simulink model "ES105A_StHlthSigNormn"  (R2013b)
settings: Solver=FixedStepDiscrete  SolverMode=SingleTasking  StartTime=0.0  StopTime=1  FixedStep=0.002  RelTol=1e-3
undefined symbols (not defined in the file): ARCHGLBPRM_FLOATZEROTHD_ULS_F32, CurrMeasCorrlnMaxErrCurr, CURRMOTSUMDIVBYZEROPROTNVAL_AMPR_F32, DIGTQDIVBYZEROPROTNVAL_HWNWTMTR_F32, DutyCycThermProtnDutyCycFildThd, EcuTMeasRngDiagcMax, EcuTMeasRngDiagcMin, EotLrngAuthyStrtLrn, FRICESTIMNDIVBYZEROPROTNVAL_HWNWTMTR_F32, HLTH0PERC_CNT_U08, HLTH100PERC_CNT_F32, HLTH100PERC_CNT_U08, HLTH50PERC_CNT_U08, HwTqCorrlnChATraSumSetFltThd, HwTqCorrlnChBTraSumSetFltThd, HWTQIDPTSIG_CNT_U08, MOTAG2MEAS_VALMAXERR_VOLTSQD_F32, MOTAG2MEAS_VALMINERR_VOLTSQD_F32, MOTAGCORRLN_MOTAGCORRLNERRTHD_MOTREVELEC_U0P16, MotDrvDiagcErrThd, MOTPOS2DIVBYZEROPROTNVAL2_VOLTSQD_F32, MOTPOS2DIVBYZEROPROTNVAL_VOLTSQD_F32, MOTPOSNERRDIVBYZEROPROTNVAL_MOTREV_U16, MOTPOSNERRZEROTHD_MOTREV_U0P16, NtcNr1, NtcSts1, PHAVLTGDIVBYZEROPROTNVAL_NANOSEC_F32, SigQlfr1, STHLTHSCAGFAC_CNT_F32, StHlthSigNormnAbsltMotPosDifStHlthDiagThd, StHlthSigNormnCurrMotSumStHlthDiagThd, StHlthSigNormnDigTqStHlthDiagThd, StHlthSigNormnDutyCycFltLimThd, StHlthSigNormnHiCtrlrT, StHlthSigNormnIdptSigStHlthSca, StHlthSigNormnLoCtrlrT, StHlthSigNormnMaxFricThd, StHlthSigNormnMinRackTrvlLim, StHlthSigNormnMotPosStHlthDiagThd, StHlthSigNormnMotVelCal, StHlthSigNormnPhaInfoStHlthDiagThd, StHlthSigNormnStHlthCorrlnErr, StHlthSigNormnStHlthCurrMotSum, StHlthSigNormnStHlthPhaInfo, StHlthSigNormnValMaxStHlthErr, StHlthSigNormnValMinStHlthErr, StHlthSigNormnWhlImbRejctnThd, SysGlbPrmMotPoleCnt, TSTHLTH0PERC_CNT_U08, u2, u3, u4, VLTGSTHLTH0PERC_CNT_U08
libraries: NxtrLim x39, simulink x33, NxtrAbslt x4
(part 2 of 10)

== system ES105A_StHlthSigNormn/StHlthSigNormn/StHlthSigNormnInit1/Motror Angle Threshold Calc ==
  note: MotAgCorrlnErrThd_p32
  note: p16
  note: p0
  note: 2^16 is max resolution
      | of 1/MotPoleCnt that won't
      | overflow u32
  note: MotPoleCnt.Max = 12
      | MotPoleCnt.Min = 2
  note: The MotAgA vs MotAgB comparison diagnostic
      | in this FDD compares MotAg signals in MotRev.
      | The safety consideration for these comparisons
      | is in MotRevElec.  Therefore the error threshold
      | has to be converted to MotRev via the following
      | relationship:
      |
      | MotRev * Np/2 = MotElec
      | MotRevElec * 2/Np = MotRev
  note: 1/MotPole_p16.Max = 32768
      | 1/MotPole_p16.Min = 5461
  note: 1 as p16
  note: MotAgCorrlnErrThd_p16
  1 as 2^16 : Constant  OutDataTypeStr=uint32
  CopyRight2 : Subsystem  Description=|  mask(Copyright Information){none=on}
      | Copyright info block.                                               
      |                                                                     
      | Place copyright information at the top of every subsystem in design.
      mask prompts: none "No parameters"
      mask help: Place copyright information at the top of every subsystem in design.
      mask Display:
      | NxtrConf = 'Nexteer Confidential';
      | 
      | sys = bdroot; %handle for the current model ("system")
      | first = get_param(sys,'Created');
      | if(isempty(first))
      |     first = datestr(now,'yyyy');
      | else
      |     first = first(end-3:end);  %year is last four digits
      | end
      | 
      | last = get_param(sys,'LastModifiedDate');
      | if isempty(last)
      |     last = datestr(now,'yyyy');
      | else
      |     last = last(end-3:end);
      | end
      | 
      | if strcmp(first,last)
      |     fprintf('%s -- Copyright %s Nexteer',NxtrConf,first)
      | else
      |     fprintf('%s -- %s%s- %s Nexteer',NxtrConf,char(169),first,last)
      | end
  Data Type Conversion{,1..4} (5 alike) : DataTypeConversion  OutDataTypeStr=uint32
  Data Type Conversion5 : DataTypeConversion  OutDataTypeStr=uint16
  Divide : Product  Inputs=*/
  Gain : Gain  Gain=-1  OutDataTypeStr=int8
  MOTAGCORRLNERRTHD_MOTREVELEC_U0P16 Data Type Max = 65535 : Constant  Value=MOTAGCORRLN_MOTAGCORRLNERRTHD_MOTREVELEC_U0P16
  MotAgCorrlnErrThd : DataStoreWrite  DataStoreName=MotAgCorrlnErrThd
  Numerator Precision : Constant  Value=16  OutDataTypeStr=int8
  Product : Product  Inputs=3
  Shift Arithmetic : ArithShift  BitShiftNumberSource=Input port  BitShiftNumber=16
      settings: InputPortMap=u0,p1
  Shift Arithmetic1 : ArithShift  BitShiftNumberSource=Input port  BitShiftNumber=16
      settings: InputPortMap=u0,p1
  SysGlbPrmMotPoleCnt : Constant  Value=SysGlbPrmMotPoleCnt
  Two Max = 2 : Constant  Value=2  OutDataTypeStr=uint32
  wires:
  SysGlbPrmMotPoleCnt/1 -> Data Type Conversion/1
  1 as 2^16/1 -> Shift Arithmetic1/1
  Shift Arithmetic1/1 -> Data Type Conversion1/1
  Data Type Conversion/1 -> Divide/2
  MOTAGCORRLNERRTHD_MOTREVELEC_U0P16 Data Type Max = 65535/1 -> Data Type Conversion2/1
  Two Max = 2/1 -> Data Type Conversion3/1
  Divide/1 -> Product/3
  Product/1 -> Data Type Conversion4/1
  Data Type Conversion3/1 -> Product/2
  Data Type Conversion2/1 -> Product/1
  Data Type Conversion5/1 -> MotAgCorrlnErrThd/1
  Data Type Conversion4/1 -> Shift Arithmetic/1
  Shift Arithmetic/1 -> Data Type Conversion5/1
  Numerator Precision/1 -> Gain/1, Shift Arithmetic/2
  Gain/1 -> Shift Arithmetic1/2
  Data Type Conversion1/1 -> Divide/1

== system ES105A_StHlthSigNormn/StHlthSigNormn/UpdRawSig/ EOT Impact Counter ==
  "HwAuthy " : Inport
  HwAg : Inport  Port=2
  RackLimrEotSig1Avl : Inport  Port=3
  HwAgEotCw : Inport  Port=4
  MotVelCrf : Inport  Port=5
  RackLimrEotSig0Avl : Inport  Port=6
  HwAgEotCcw : Inport  Port=7
  "Case:{}" : ActionPort  ActionType=case
  Constant : Constant  Value=EotLrngAuthyStrtLrn
  CopyRight2 : Subsystem  Description=|  mask(Copyright Information){none=on}
      | Copyright info block.                                               
      |                                                                     
      | Place copyright information at the top of every subsystem in design.
      mask prompts: none "No parameters"
      mask help: Place copyright information at the top of every subsystem in design.
      mask Display:
      | NxtrConf = 'Nexteer Confidential';
      | 
      | sys = bdroot; %handle for the current model ("system")
      | first = get_param(sys,'Created');
      | first = first(end-3:end);  %year is last four digits
      | 
      | last = get_param(sys,'LastModifiedDate');
      | if isempty(last)
      |     last = datestr(now,'yyyy');
      | else
      |     last = last(end-3:end);
      | end
      | 
      | if strcmp(first,last)
      |     fprintf('%s -- Copyright %s Nexteer',NxtrConf,first)
      | else
      |     fprintf('%s -- %s%s- %s Nexteer',NxtrConf,char(169),first,last)
      | end
  Data Store Read : DataStoreRead  DataStoreName=EotImpctCntr
  If : If  IfExpression=u1
  If Action Subsystem : Subsystem  TreatAsAtomicUnit=on
  If Action Subsystem1 : Subsystem  TreatAsAtomicUnit=on
  LimStat_u2 : NxtrLim/LimStat_u08  LoLim=EotImpctStHlth.EngMin  HiLim=EotImpctStHlth.EngMax
      settings: AttributesFormatString=|
      | Low Limit: %<LoLim>
      | High Limit:%<HiLim>
  Relational Operator : RelationalOperator  Operator=>  OutDataTypeStr=boolean
  EotImpctStHlth : Outport
  wires:
  "HwAuthy "/1 -> Relational Operator/1
  Constant/1 -> Relational Operator/2
  Relational Operator/1 -> If/1
  If/1 -> If Action Subsystem/Action
  HwAg/1 -> If Action Subsystem/1(HwAg)
  If/2 -> If Action Subsystem1/Action
  RackLimrEotSig1Avl/1 -> If Action Subsystem/5(RackLimrEotSig1Avl)
  RackLimrEotSig0Avl/1 -> If Action Subsystem/2(RackLimrEotSig0Avl)
  HwAgEotCw/1 -> If Action Subsystem/6(HwAgEotCw)
  MotVelCrf/1 -> If Action Subsystem/3(MotVelCrf)
  HwAgEotCcw/1 -> If Action Subsystem/4(HwAgEotCcw)
  Data Store Read/1 -> LimStat_u2/1
  LimStat_u2/1 -> EotImpctStHlth/1

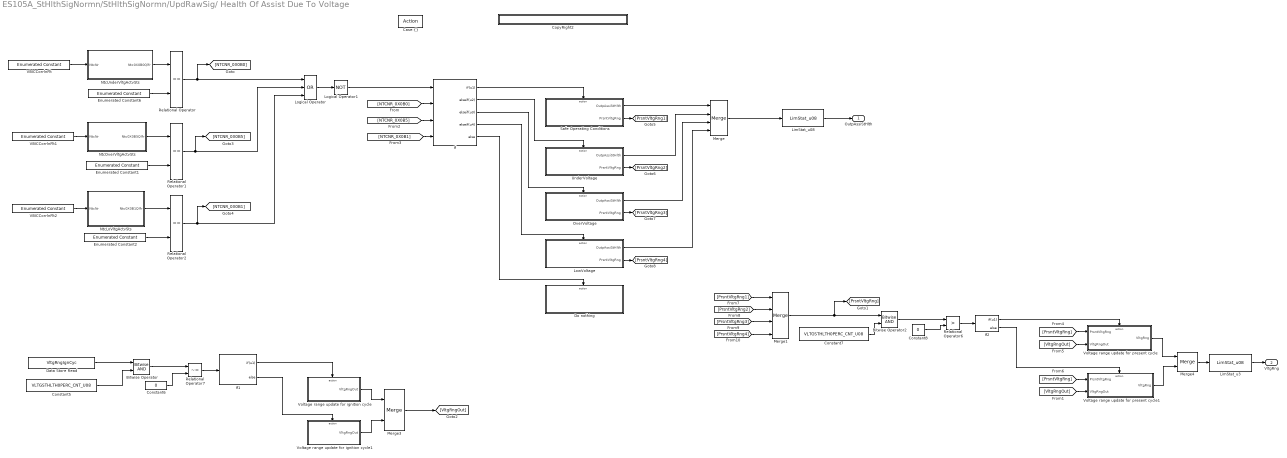
== system ES105A_StHlthSigNormn/StHlthSigNormn/UpdRawSig/ Health Of Assist Due To Voltage ==
  "Case:{}" : ActionPort  ActionType=case
  Bitwise Operator : simulink/Logic and Bit Operations/Bitwise Operator  logicop=AND  UseBitMask=off  NumInputPorts=2  BitMask=bin2dec('11011001')  BitMaskRealWorld=Stored Integer
  Bitwise Operator2 : simulink/Logic and Bit Operations/Bitwise Operator  logicop=AND  UseBitMask=off  NumInputPorts=2  BitMask=bin2dec('11011001')  BitMaskRealWorld=Stored Integer
  Constant5 : Constant  Value=VLTGSTHLTH0PERC_CNT_U08
  Constant6 : Constant  Value=0  OutDataTypeStr=uint8
      settings: AttributesFormatString=%<OutDataTypeStr>
  Constant7 : Constant  Value=VLTGSTHLTH0PERC_CNT_U08
  Constant8 : Constant  Value=0  OutDataTypeStr=uint8
      settings: AttributesFormatString=%<OutDataTypeStr>
  CopyRight2 : Subsystem  Description=|  mask(Copyright Information){none=on}
      | Copyright info block.                                               
      |                                                                     
      | Place copyright information at the top of every subsystem in design.
      mask prompts: none "No parameters"
      mask help: Place copyright information at the top of every subsystem in design.
      mask Display:
      | NxtrConf = 'Nexteer Confidential';
      | 
      | sys = bdroot; %handle for the current model ("system")
      | first = get_param(sys,'Created');
      | first = first(end-3:end);  %year is last four digits
      | 
      | last = get_param(sys,'LastModifiedDate');
      | if isempty(last)
      |     last = datestr(now,'yyyy');
      | else
      |     last = last(end-3:end);
      | end
      | 
      | if strcmp(first,last)
      |     fprintf('%s -- Copyright %s Nexteer',NxtrConf,first)
      | else
      |     fprintf('%s -- %s%s- %s Nexteer',NxtrConf,char(169),first,last)
      | end
  Data Store Read : DataStoreRead  DataStoreName=VltgRngIgnCyc
  Do nothing : Subsystem
  Enumerated Constant1 : simulink/Sources/Enumerated Constant  OutDataTypeStr=Enum: SigQlfr1  Value=SigQlfr1.SIGQLFR_FAILD  SampleTime=inf
  Enumerated Constant2 : simulink/Sources/Enumerated Constant  OutDataTypeStr=Enum: SigQlfr1  Value=SigQlfr1.SIGQLFR_FAILD  SampleTime=inf
  Enumerated Constant6 : simulink/Sources/Enumerated Constant  OutDataTypeStr=Enum: SigQlfr1  Value=SigQlfr1.SIGQLFR_FAILD  SampleTime=inf
  If : If  NumInputs=4  IfExpression=u1  ElseIfExpressions=u2,u3,u4
  If1 : If  IfExpression=u1
  If2 : If  IfExpression=u1
  LimStat_u08 : NxtrLim/LimStat_u08  LoLim=OutpAssiStHlth.EngMin  HiLim=OutpAssiStHlth.EngMax
      settings: AttributesFormatString=|
      | Low Limit: %<LoLim>
      | High Limit:%<HiLim>
  LimStat_u3 : NxtrLim/LimStat_u08  LoLim=VltgRng.EngMin  HiLim=VltgRng.EngMax
      settings: AttributesFormatString=|
      | Low Limit: %<LoLim>
      | High Limit:%<HiLim>
  Logical Operator : Logic  RequirementInfo={'linktype_rmi_doors' '0001022c (/ESG Group/FDD Module Requirements/EA4 Specific/ES105A_StHlthSigNormn)' '#ES105A_50' 'true' 'REQ: ES105A_50' '' } %GIDa_9a5ea61a_ea12_4910_a0fe_06a0e1905550  Operator=OR  Inputs=3  AllPortsSameDT=off  OutDataTypeStr=boolean
  Logical Operator1 : Logic  RequirementInfo={'linktype_rmi_doors' '0001022c (/ESG Group/FDD Module Requirements/EA4 Specific/ES105A_StHlthSigNormn)' '#ES105A_50' 'true' 'REQ: ES105A_50' '' } %GIDa_f3dc77f5_d391_4300_bddf_a50a41924f40  Operator=NOT  AllPortsSameDT=off  OutDataTypeStr=boolean
  LowVoltage : Subsystem  RequirementInfo={'linktype_rmi_doors' '0001022c (/ESG Group/FDD Module Requirements/EA4 Specific/ES105A_StHlthSigNormn)' '#ES105A_53' 'true' 'REQ: ES105A_53' '' } %GIDa_506e871b_8543_4634_a577_67c158e429f9
  Merge : Merge  Inputs=4
  Merge1 : Merge  Inputs=4
  Merge3 : Merge
  Merge4 : Merge
  NtcLoVltgActvSts : Subsystem  RequirementInfo={} %GIDa_d5ea79d0_4b56_4532_81dc_37f5b337e086  TreatAsAtomicUnit=on  mask(GetNTC){}
      mask help: GetNTC library block
      settings: RTWSystemCode=Inline
  NtcOverVltgActvSts : Subsystem  RequirementInfo={} %GIDa_e1e8ebde_c4f9_4f8d_a1e3_0543f63840ce  TreatAsAtomicUnit=on  mask(GetNTC){}
      mask help: GetNTC library block
      settings: RTWSystemCode=Inline
  NtcUnderVltgActvSts : Subsystem  RequirementInfo={} %GIDa_9b87baab_3980_45fe_8d54_a3baaaee6b6f  TreatAsAtomicUnit=on  mask(GetNTC){}
      mask help: GetNTC library block
      settings: RTWSystemCode=Inline
  OverVoltage : Subsystem  RequirementInfo={'linktype_rmi_doors' '0001022c (/ESG Group/FDD Module Requirements/EA4 Specific/ES105A_StHlthSigNormn)' '#ES105A_52' 'true' 'REQ: ES105A_52' '' } %GIDa_cd3c8530_bf41_482a_97a1_1e49fef579f6
  Relational Operator : RelationalOperator  Operator===  OutDataTypeStr=boolean
  Relational Operator1 : RelationalOperator  Operator===  OutDataTypeStr=boolean
  Relational Operator2 : RelationalOperator  Operator===  OutDataTypeStr=boolean
  Relational Operator6 : RelationalOperator  Operator=>  OutDataTypeStr=boolean
  Relational Operator7 : RelationalOperator  Operator=~=  OutDataTypeStr=boolean
  Safe Operating Conditions : Subsystem  RequirementInfo={'linktype_rmi_doors' '0001022c (/ESG Group/FDD Module Requirements/EA4 Specific/ES105A_StHlthSigNormn)' '#ES105A_50' 'true' 'REQ: ES105A_50' '' } %GIDa_08090837_8a60_4bda_aaf5_7b407a469d1b
  UnderVoltage : Subsystem  RequirementInfo={'linktype_rmi_doors' '0001022c (/ESG Group/FDD Module Requirements/EA4 Specific/ES105A_StHlthSigNormn)' '#ES105A_51' 'true' 'REQ: ES105A_51' '' } %GIDa_8bbe1a5e_3828_4897_9c76_848f46c9da8f
  VBICCorrlnFlt : simulink/Sources/Enumerated Constant  RequirementInfo={'linktype_rmi_doors' '0001022c (/ESG Group/FDD Module Requirements/EA4 Specific/ES105A_StHlthSigNormn)' '#ES105A_15' 'true' 'REQ: ES105A_15' '' } %GIDa_abcae5bb_89f4_46e7_b061_adbd8ff599e2  OutDataTypeStr=Enum: NtcNr1  Value=NtcNr1.NTCNR_0X0B0  SampleTime=inf
  VBICCorrlnFlt1 : simulink/Sources/Enumerated Constant  RequirementInfo={'linktype_rmi_doors' '0001022c (/ESG Group/FDD Module Requirements/EA4 Specific/ES105A_StHlthSigNormn)' '#ES105A_15' 'true' 'REQ: ES105A_15' '' } %GIDa_5d58c9da_5328_4e21_8197_5deed1f7c707  OutDataTypeStr=Enum: NtcNr1  Value=NtcNr1.NTCNR_0X0B5  SampleTime=inf
  VBICCorrlnFlt2 : simulink/Sources/Enumerated Constant  RequirementInfo={'linktype_rmi_doors' '0001022c (/ESG Group/FDD Module Requirements/EA4 Specific/ES105A_StHlthSigNormn)' '#ES105A_15' 'true' 'REQ: ES105A_15' '' } %GIDa_7ebd8b39_32ce_4267_96b1_a79cedaf356f  OutDataTypeStr=Enum: NtcNr1  Value=NtcNr1.NTCNR_0X0B1  SampleTime=inf
  Voltage range update for ignition cycle : Subsystem  RequirementInfo={'linktype_rmi_doors' '0001022c (/ESG Group/FDD Module Requirements/EA4 Specific/ES105A_StHlthSigNormn)' '#ES105A_54' 'true' 'REQ: ES105A_54' '' } %GIDa_370b8f01_3508_495b_a218_3f1e9e3ef072  TreatAsAtomicUnit=on
  Voltage range update for ignition cycle1 : Subsystem  RequirementInfo={'linktype_rmi_doors' '0001022c (/ESG Group/FDD Module Requirements/EA4 Specific/ES105A_StHlthSigNormn)' '#ES105A_54' 'true' 'REQ: ES105A_54' '' } %GIDa_2af8c5ef_4773_490c_9b01_2c7f0f74e411  TreatAsAtomicUnit=on
  "Voltage range update for present cycle " : Subsystem  RequirementInfo={'linktype_rmi_doors' '0001022c (/ESG Group/FDD Module Requirements/EA4 Specific/ES105A_StHlthSigNormn)' '#ES105A_54' 'true' 'REQ: ES105A_54' '' } %GIDa_0b645a7d_a4a8_4e36_bf1f_844e4b7dab81  TreatAsAtomicUnit=on
  Voltage range update for present cycle1 : Subsystem  RequirementInfo={'linktype_rmi_doors' '0001022c (/ESG Group/FDD Module Requirements/EA4 Specific/ES105A_StHlthSigNormn)' '#ES105A_54' 'true' 'REQ: ES105A_54' '' } %GIDa_a391510e_bc04_4784_82e4_9c19ec1d09bb  TreatAsAtomicUnit=on
  OutpAssiStHlth : Outport
  " VltgRng" : Outport  Port=2
  wires:
  NtcUnderVltgActvSts/1(Ntc0X0B0Qlfr) -> Relational Operator/1
  Enumerated Constant6/1 -> Relational Operator/2
  VBICCorrlnFlt/1 -> NtcUnderVltgActvSts/1(NtcNr)
  VBICCorrlnFlt1/1 -> NtcOverVltgActvSts/1(NtcNr)
  VBICCorrlnFlt2/1 -> NtcLoVltgActvSts/1(NtcNr)
  NtcOverVltgActvSts/1(Ntc0X0B5Qlfr) -> Relational Operator1/1
  Enumerated Constant1/1 -> Relational Operator1/2
  NtcLoVltgActvSts/1(Ntc0X0B1Qlfr) -> Relational Operator2/1
  Enumerated Constant2/1 -> Relational Operator2/2
  Logical Operator/1 -> Logical Operator1/1
  Constant8/1 -> Relational Operator6/2
  Relational Operator6/1 -> If2/1
  If2/1 -> "Voltage range update for present cycle "/Action
  If2/2 -> Voltage range update for present cycle1/Action
  [PrsntVltgRng] -> "Voltage range update for present cycle "/1(PrsntVltgRng)
  [VltgRngOut] -> "Voltage range update for present cycle "/2(VltgRngOut)
  Bitwise Operator2/1 -> Relational Operator6/1
  [PrsntVltgRng] -> Voltage range update for present cycle1/1(PrsntVltgRng)
  Constant6/1 -> Relational Operator7/2
  Relational Operator7/1 -> If1/1
  If1/1 -> Voltage range update for ignition cycle/Action
  Voltage range update for ignition cycle/1(VltgRngOut) -> Merge3/1
  Voltage range update for ignition cycle1/1(VltgRngOut) -> Merge3/2
  Data Store Read/1 -> Bitwise Operator/1
  Constant5/1 -> Bitwise Operator/2
  Bitwise Operator/1 -> Relational Operator7/1
  [VltgRngOut] -> Voltage range update for present cycle1/2(VltgRngOut)
  Merge3/1 -> [VltgRngOut]
  [NTCNR_0X0B0] -> If/2
  [NTCNR_0X0B5] -> If/3
  [NTCNR_0X0B1] -> If/4
  Merge1/1 -> [PrsntVltgRng], Bitwise Operator2/1
  "Voltage range update for present cycle "/1(" VltgRng") -> Merge4/1
  Voltage range update for present cycle1/1(" VltgRng") -> Merge4/2
  If1/2 -> Voltage range update for ignition cycle1/Action
  If/1 -> Safe Operating Conditions/Action
  If/2 -> UnderVoltage/Action
  If/3 -> OverVoltage/Action
  If/4 -> LowVoltage/Action
  If/5 -> Do nothing/Action
  Safe Operating Conditions/1(OutpAssiStHlth) -> Merge/1
  UnderVoltage/1(OutpAssiStHlth) -> Merge/2
  OverVoltage/1(OutpAssiStHlth) -> Merge/3
  LowVoltage/1(OutpAssiStHlth) -> Merge/4
  Relational Operator1/1 -> [NTCNR_0X0B5], Logical Operator/2
  Safe Operating Conditions/2(" PrsntVltgRng") -> [PrsntVltgRng1]
  UnderVoltage/2(" PrsntVltgRng") -> [PrsntVltgRng2]
  OverVoltage/2(" PrsntVltgRng") -> [PrsntVltgRng3]
  LowVoltage/2(" PrsntVltgRng") -> [PrsntVltgRng4]
  [PrsntVltgRng1] -> Merge1/1
  [PrsntVltgRng2] -> Merge1/2
  [PrsntVltgRng3] -> Merge1/3
  [PrsntVltgRng4] -> Merge1/4
  Constant7/1 -> Bitwise Operator2/2
  Relational Operator2/1 -> [NTCNR_0X0B1], Logical Operator/3
  Relational Operator/1 -> [NTCNR_0X0B0], Logical Operator/1
  Logical Operator1/1 -> If/1
  Merge/1 -> LimStat_u08/1
  Merge4/1 -> LimStat_u3/1
  LimStat_u08/1 -> OutpAssiStHlth/1
  LimStat_u3/1 -> " VltgRng"/1

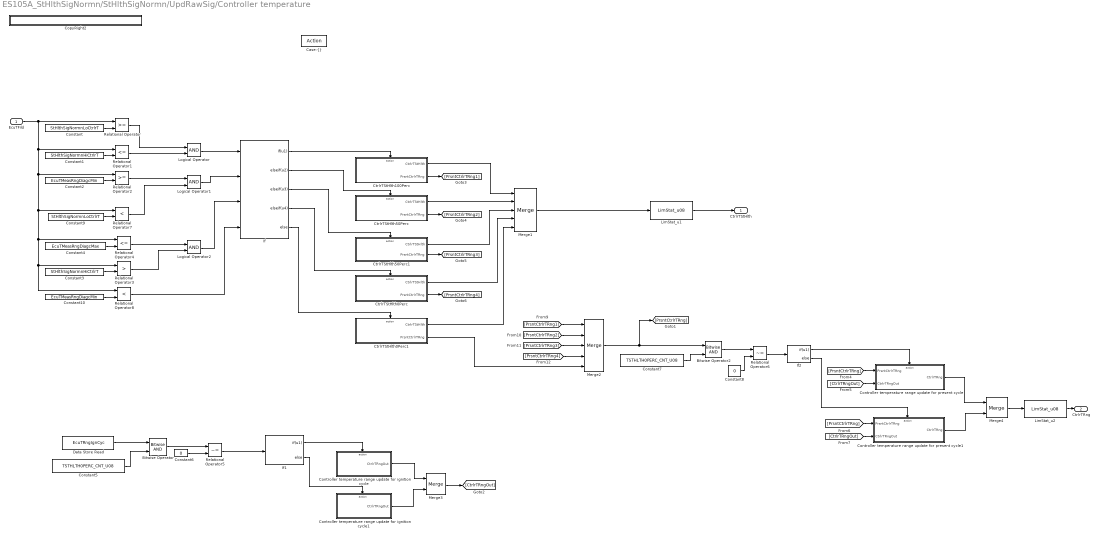
== system ES105A_StHlthSigNormn/StHlthSigNormn/UpdRawSig/Controller temperature ==
  EcuTFild : Inport
  "Case:{}" : ActionPort  ActionType=case
  Bitwise Operator : simulink/Logic and Bit Operations/Bitwise Operator  logicop=AND  UseBitMask=off  NumInputPorts=2  BitMask=bin2dec('11011001')  BitMaskRealWorld=Stored Integer
  Bitwise Operator2 : simulink/Logic and Bit Operations/Bitwise Operator  logicop=AND  UseBitMask=off  NumInputPorts=2  BitMask=bin2dec('11011001')  BitMaskRealWorld=Stored Integer
  Constant : Constant  Value=StHlthSigNormnLoCtrlrT
  Constant1 : Constant  Value=StHlthSigNormnHiCtrlrT
  Constant10 : Constant  Value=EcuTMeasRngDiagcMin
  Constant2 : Constant  Value=EcuTMeasRngDiagcMin
  Constant3 : Constant  Value=StHlthSigNormnHiCtrlrT
  Constant4 : Constant  Value=EcuTMeasRngDiagcMax
  Constant5 : Constant  Value=TSTHLTH0PERC_CNT_U08
  Constant6 : Constant  Value=0  OutDataTypeStr=uint8
      settings: AttributesFormatString=%<OutDataTypeStr>
  Constant7 : Constant  Value=TSTHLTH0PERC_CNT_U08
  Constant8 : Constant  Value=0  OutDataTypeStr=uint8
      settings: AttributesFormatString=%<OutDataTypeStr>
  Constant9 : Constant  Value=StHlthSigNormnLoCtrlrT
  Controller temperature range update for ignition cycle : Subsystem  RequirementInfo={'linktype_rmi_doors' '0001022c (/ESG Group/FDD Module Requirements/EA4 Specific/ES105A_StHlthSigNormn)' '#ES105A_46' 'true' 'REQ: ES105A_46' '' } %GIDa_ba23833c_117c_41a7_aecf_6cb2bb29f491  TreatAsAtomicUnit=on
  Controller temperature range update for ignition cycle1 : Subsystem  RequirementInfo={'linktype_rmi_doors' '0001022c (/ESG Group/FDD Module Requirements/EA4 Specific/ES105A_StHlthSigNormn)' '#ES105A_46' 'true' 'REQ: ES105A_46' '' } %GIDa_15dd9d5b_80e5_4058_b203_7867af7ff412  TreatAsAtomicUnit=on
  "Controller temperature range update for present cycle " : Subsystem  RequirementInfo={'linktype_rmi_doors' '0001022c (/ESG Group/FDD Module Requirements/EA4 Specific/ES105A_StHlthSigNormn)' '#ES105A_46' 'true' 'REQ: ES105A_46' '' } %GIDa_f109f1a5_b605_4805_b7e1_315c1ae60bf3  TreatAsAtomicUnit=on
  Controller temperature range update for present cycle1 : Subsystem  RequirementInfo={'linktype_rmi_doors' '0001022c (/ESG Group/FDD Module Requirements/EA4 Specific/ES105A_StHlthSigNormn)' '#ES105A_46' 'true' 'REQ: ES105A_46' '' } %GIDa_66754047_f90b_435e_b357_765d1592d9e2  TreatAsAtomicUnit=on
  CopyRight2 : Subsystem  Description=|  mask(Copyright Information){none=on}
      | Copyright info block.                                               
      |                                                                     
      | Place copyright information at the top of every subsystem in design.
      mask prompts: none "No parameters"
      mask help: Place copyright information at the top of every subsystem in design.
      mask Display:
      | NxtrConf = 'Nexteer Confidential';
      | 
      | sys = bdroot; %handle for the current model ("system")
      | first = get_param(sys,'Created');
      | first = first(end-3:end);  %year is last four digits
      | 
      | last = get_param(sys,'LastModifiedDate');
      | if isempty(last)
      |     last = datestr(now,'yyyy');
      | else
      |     last = last(end-3:end);
      | end
      | 
      | if strcmp(first,last)
      |     fprintf('%s -- Copyright %s Nexteer',NxtrConf,first)
      | else
      |     fprintf('%s -- %s%s- %s Nexteer',NxtrConf,char(169),first,last)
      | end
  CtrlrTStHlth0Perc : Subsystem  RequirementInfo={'linktype_rmi_doors' '0001022c (/ESG Group/FDD Module Requirements/EA4 Specific/ES105A_StHlthSigNormn)' '#ES105A_44' 'true' 'REQ: ES105A_44' '' ; 'linktype_rmi_doors' '0001022c (/ESG Group/FDD Module Requirements/EA4 Specific/ES105A_StHlthSigNormn)' '#ES105A_46' 'true' 'REQ: ES105A_46' '' } %GIDa_bc23de3d_cc5d_48c0_85bb_1f30533f593a  TreatAsAtomicUnit=on
  CtrlrTStHlth0Perc1 : Subsystem  RequirementInfo={'linktype_rmi_doors' '0001022c (/ESG Group/FDD Module Requirements/EA4 Specific/ES105A_StHlthSigNormn)' '#ES105A_45' 'true' 'REQ: ES105A_45' '' ; 'linktype_rmi_doors' '0001022c (/ESG Group/FDD Module Requirements/EA4 Specific/ES105A_StHlthSigNormn)' '#ES105A_46' 'true' 'REQ: ES105A_46' '' } %GIDa_a6f1872e_abef_47a2_ac8a_186dbaa520a0  TreatAsAtomicUnit=on
  CtrlrTStHlth100Perc : Subsystem  RequirementInfo={'linktype_rmi_doors' '0001022c (/ESG Group/FDD Module Requirements/EA4 Specific/ES105A_StHlthSigNormn)' '#ES105A_41' 'true' 'REQ: ES105A_41' '' ; 'linktype_rmi_doors' '0001022c (/ESG Group/FDD Module Requirements/EA4 Specific/ES105A_StHlthSigNormn)' '#ES105A_46' 'true' 'REQ: ES105A_46' '' } %GIDa_13e6b6a8_a03c_4c8e_a328_837a68683571  TreatAsAtomicUnit=on
  CtrlrTStHlth50Perc : Subsystem  RequirementInfo={'linktype_rmi_doors' '0001022c (/ESG Group/FDD Module Requirements/EA4 Specific/ES105A_StHlthSigNormn)' '#ES105A_42' 'true' 'REQ: ES105A_42' '' ; 'linktype_rmi_doors' '0001022c (/ESG Group/FDD Module Requirements/EA4 Specific/ES105A_StHlthSigNormn)' '#ES105A_46' 'true' 'REQ: ES105A_46' '' } %GIDa_98ca9737_9799_40d9_9f48_42638f292199  TreatAsAtomicUnit=on
  CtrlrTStHlth50Perc1 : Subsystem  RequirementInfo={'linktype_rmi_doors' '0001022c (/ESG Group/FDD Module Requirements/EA4 Specific/ES105A_StHlthSigNormn)' '#ES105A_43' 'true' 'REQ: ES105A_43' '' ; 'linktype_rmi_doors' '0001022c (/ESG Group/FDD Module Requirements/EA4 Specific/ES105A_StHlthSigNormn)' '#ES105A_46' 'true' 'REQ: ES105A_46' '' } %GIDa_2817e139_7daa_4e54_bfe4_0a17f88bfe20  TreatAsAtomicUnit=on
  Data Store Read : DataStoreRead  DataStoreName=EcuTRngIgnCyc
  If : If  NumInputs=4  IfExpression=u1  ElseIfExpressions=u2,u3,u4
  If1 : If  IfExpression=u1
  If2 : If  IfExpression=u1
  LimStat_u1 : NxtrLim/LimStat_u08  LoLim=CtrlrTStHlth.EngMin  HiLim=CtrlrTStHlth.EngMax
      settings: AttributesFormatString=|
      | Low Limit: %<LoLim>
      | High Limit:%<HiLim>
  LimStat_u2 : NxtrLim/LimStat_u08  LoLim=CtrlrTRng.EngMin  HiLim=CtrlrTRng.EngMax
      settings: AttributesFormatString=|
      | Low Limit: %<LoLim>
      | High Limit:%<HiLim>
  Logical Operator : Logic  AllPortsSameDT=off  OutDataTypeStr=boolean
  Logical Operator1 : Logic  AllPortsSameDT=off  OutDataTypeStr=boolean
  Logical Operator2 : Logic  AllPortsSameDT=off  OutDataTypeStr=boolean
  Merge1 : Merge  Inputs=5
  Merge2 : Merge  Inputs=5
  Merge3 : Merge
  Merge4 : Merge
  Relational Operator : RelationalOperator  RequirementInfo={'linktype_rmi_doors' '0001022c (/ESG Group/FDD Module Requirements/EA4 Specific/ES105A_StHlthSigNormn)' '#ES105A_41' 'true' 'REQ: ES105A_41' '' } %GIDa_37ea3b07_d616_4d9d_9c23_e05da49f2996  OutDataTypeStr=boolean
  Relational Operator1 : RelationalOperator  RequirementInfo={'linktype_rmi_doors' '0001022c (/ESG Group/FDD Module Requirements/EA4 Specific/ES105A_StHlthSigNormn)' '#ES105A_41' 'true' 'REQ: ES105A_41' '' } %GIDa_62cba185_5b8e_40d0_bd60_bab0077a1c8f  Operator=<=  OutDataTypeStr=boolean
  Relational Operator2 : RelationalOperator  RequirementInfo={'linktype_rmi_doors' '0001022c (/ESG Group/FDD Module Requirements/EA4 Specific/ES105A_StHlthSigNormn)' '#ES105A_42' 'true' 'REQ: ES105A_42' '' } %GIDa_355f0303_7889_4320_8a8f_69a6bfdd2b65  OutDataTypeStr=boolean
  Relational Operator3 : RelationalOperator  RequirementInfo={'linktype_rmi_doors' '0001022c (/ESG Group/FDD Module Requirements/EA4 Specific/ES105A_StHlthSigNormn)' '#ES105A_43' 'true' 'REQ: ES105A_43' '' } %GIDa_8020b49f_98e9_4fb3_890f_9983d7a60b03  Operator=>  OutDataTypeStr=boolean
  Relational Operator4 : RelationalOperator  RequirementInfo={'linktype_rmi_doors' '0001022c (/ESG Group/FDD Module Requirements/EA4 Specific/ES105A_StHlthSigNormn)' '#ES105A_43' 'true' 'REQ: ES105A_43' '' } %GIDa_1c0f9b03_3041_4a07_b447_f5c399357400  Operator=<=  OutDataTypeStr=boolean
  Relational Operator5 : RelationalOperator  Operator=~=  OutDataTypeStr=boolean
  Relational Operator6 : RelationalOperator  Operator=~=  OutDataTypeStr=boolean
  Relational Operator7 : RelationalOperator  RequirementInfo={'linktype_rmi_doors' '0001022c (/ESG Group/FDD Module Requirements/EA4 Specific/ES105A_StHlthSigNormn)' '#ES105A_42' 'true' 'REQ: ES105A_42' '' } %GIDa_f158360d_efc3_43a0_8245_87bd8d25bb6c  Operator=<  OutDataTypeStr=boolean
  Relational Operator8 : RelationalOperator  RequirementInfo={'linktype_rmi_doors' '0001022c (/ESG Group/FDD Module Requirements/EA4 Specific/ES105A_StHlthSigNormn)' '#ES105A_44' 'true' 'REQ: ES105A_44' '' } %GIDa_14ade3ec_9658_43c4_a9bf_48634e6a9bd8  Operator=<  OutDataTypeStr=boolean
  CtrlrTStHlth : Outport
  CtrlrTRng : Outport  Port=2
  wires:
  Constant/1 -> Relational Operator/2
  Constant1/1 -> Relational Operator1/2
  Relational Operator/1 -> Logical Operator/1
  Relational Operator1/1 -> Logical Operator/2
  Logical Operator/1 -> If/1
  Constant2/1 -> Relational Operator2/2
  EcuTFild/1 -> Relational Operator4/1, Relational Operator3/1, Relational Operator8/1, Relational Operator7/1, Relational Operator2/1, Relational Operator1/1, Relational Operator/1
  Constant4/1 -> Relational Operator4/2
  CtrlrTStHlth100Perc/1(CtrlrTStHlth) -> Merge1/1
  If/1 -> CtrlrTStHlth100Perc/Action
  If/2 -> CtrlrTStHlth50Perc/Action
  Constant6/1 -> Relational Operator5/2
  Relational Operator5/1 -> If1/1
  If1/1 -> Controller temperature range update for ignition cycle/Action
  If1/2 -> Controller temperature range update for ignition cycle1/Action
  Controller temperature range update for ignition cycle1/1(CtrlrTRngOut) -> Merge3/2
  Merge3/1 -> [CtrlrTRngOut]
  Constant8/1 -> Relational Operator6/2
  If2/1 -> "Controller temperature range update for present cycle "/Action
  If2/2 -> Controller temperature range update for present cycle1/Action
  Merge2/1 -> Bitwise Operator2/1, [PrsntCtrlrTRng]
  [PrsntCtrlrTRng] -> "Controller temperature range update for present cycle "/1(PrsntCtrlrTRng)
  [CtrlrTRngOut] -> "Controller temperature range update for present cycle "/2(CtrlrTRngOut)
  Data Store Read/1 -> Bitwise Operator/1
  Constant5/1 -> Bitwise Operator/2
  Bitwise Operator/1 -> Relational Operator5/1
  Constant7/1 -> Bitwise Operator2/2
  Bitwise Operator2/1 -> Relational Operator6/1
  [PrsntCtrlrTRng] -> Controller temperature range update for present cycle1/1(PrsntCtrlrTRng)
  "Controller temperature range update for present cycle "/1(CtrlrTRng) -> Merge4/1
  Controller temperature range update for present cycle1/1(CtrlrTRng) -> Merge4/2
  CtrlrTStHlth50Perc/1(CtrlrTStHlth) -> Merge1/2
  Relational Operator6/1 -> If2/1
  [CtrlrTRngOut] -> Controller temperature range update for present cycle1/2(CtrlrTRngOut)
  Constant9/1 -> Relational Operator7/2
  Relational Operator2/1 -> Logical Operator1/1
  Relational Operator7/1 -> Logical Operator1/2
  Logical Operator1/1 -> If/2
  If/3 -> CtrlrTStHlth50Perc1/Action
  CtrlrTStHlth50Perc1/1(CtrlrTStHlth) -> Merge1/3
  CtrlrTStHlth100Perc/2(PrsntCtrlrTRng) -> [PrsntCtrlrTRng1]
  CtrlrTStHlth50Perc1/2(PrsntCtrlrTRng) -> [PrsntCtrlrTRng3]
  [PrsntCtrlrTRng1] -> Merge2/1
  [PrsntCtrlrTRng2] -> Merge2/2
  [PrsntCtrlrTRng3] -> Merge2/3
  [PrsntCtrlrTRng4] -> Merge2/4
  Controller temperature range update for ignition cycle/1(CtrlrTRngOut) -> Merge3/1
  CtrlrTStHlth50Perc/2(PrsntCtrlrTRng) -> [PrsntCtrlrTRng2]
  Constant3/1 -> Relational Operator3/2
  Relational Operator4/1 -> Logical Operator2/1
  Relational Operator3/1 -> Logical Operator2/2
  Logical Operator2/1 -> If/3
  Constant10/1 -> Relational Operator8/2
  Relational Operator8/1 -> If/4
  If/4 -> CtrlrTStHlth0Perc/Action
  If/5 -> CtrlrTStHlth0Perc1/Action
  CtrlrTStHlth0Perc/2(PrsntCtrlrTRng) -> [PrsntCtrlrTRng4]
  CtrlrTStHlth0Perc1/2(PrsntCtrlrTRng) -> Merge2/5
  CtrlrTStHlth0Perc/1(CtrlrTStHlth) -> Merge1/4
  CtrlrTStHlth0Perc1/1(CtrlrTStHlth) -> Merge1/5
  Merge1/1 -> LimStat_u1/1
  Merge4/1 -> LimStat_u2/1
  LimStat_u1/1 -> CtrlrTStHlth/1
  LimStat_u2/1 -> CtrlrTRng/1

== system ES105A_StHlthSigNormn/StHlthSigNormn/UpdRawSig/CopyRight2 ==

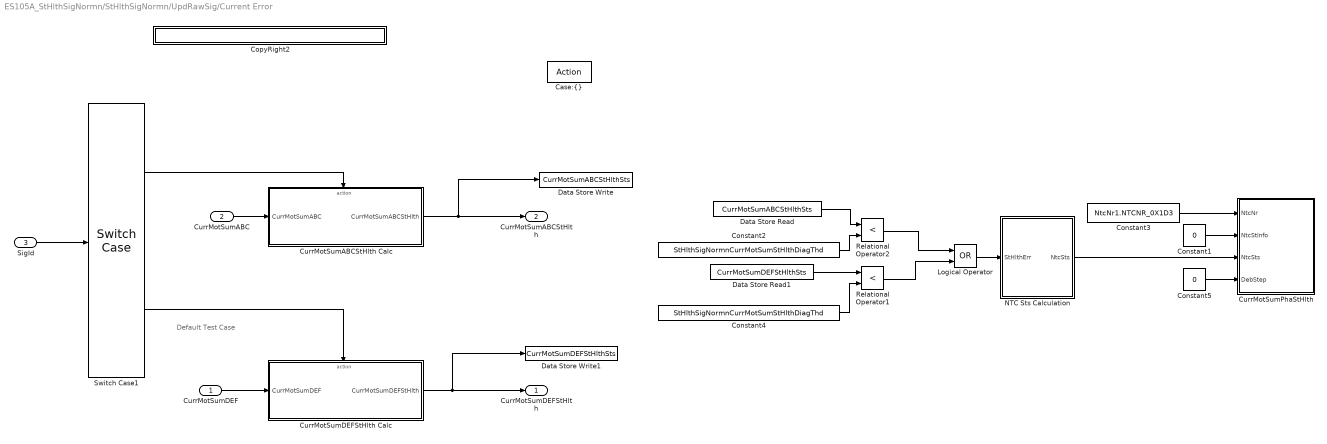
== system ES105A_StHlthSigNormn/StHlthSigNormn/UpdRawSig/Current Error ==
  note: Default Test Case
  CurrMotSumDEF : Inport
  CurrMotSumABC : Inport  Port=2
  SigId : Inport  Port=3
  "Case:{}" : ActionPort  ActionType=case
  Constant1 : Constant  Value=0  OutDataTypeStr=uint8
      settings: AttributesFormatString=%<OutDataTypeStr>
  Constant2 : Constant  Value=StHlthSigNormnCurrMotSumStHlthDiagThd
  Constant3 : Constant  Value=NtcNr1.NTCNR_0X1D3  OutDataTypeStr=Enum: NtcNr1
  Constant4 : Constant  Value=StHlthSigNormnCurrMotSumStHlthDiagThd
  Constant5 : Constant  Value=0  OutDataTypeStr=uint16
      settings: AttributesFormatString=%<OutDataTypeStr>
  CopyRight2 : Subsystem  Description=|  mask(Copyright Information){none=on}
      | Copyright info block.                                               
      |                                                                     
      | Place copyright information at the top of every subsystem in design.
      mask prompts: none "No parameters"
      mask help: Place copyright information at the top of every subsystem in design.
      mask Display:
      | NxtrConf = 'Nexteer Confidential';
      | 
      | sys = bdroot; %handle for the current model ("system")
      | first = get_param(sys,'Created');
      | first = first(end-3:end);  %year is last four digits
      | 
      | last = get_param(sys,'LastModifiedDate');
      | if isempty(last)
      |     last = datestr(now,'yyyy');
      | else
      |     last = last(end-3:end);
      | end
      | 
      | if strcmp(first,last)
      |     fprintf('%s -- Copyright %s Nexteer',NxtrConf,first)
      | else
      |     fprintf('%s -- %s%s- %s Nexteer',NxtrConf,char(169),first,last)
      | end
  CurrMotSumABCStHlth Calc : Subsystem  TreatAsAtomicUnit=on
  CurrMotSumDEFStHlth Calc : Subsystem  TreatAsAtomicUnit=on
  CurrMotSumPhaStHlth : Subsystem  mask(SetNTC){}
      mask help: SetNTC library block
  Data Store Read : DataStoreRead  DataStoreName=CurrMotSumABCStHlthSts
  Data Store Read1 : DataStoreRead  DataStoreName=CurrMotSumDEFStHlthSts
  Data Store Write : DataStoreWrite  DataStoreName=CurrMotSumABCStHlthSts
  Data Store Write1 : DataStoreWrite  DataStoreName=CurrMotSumDEFStHlthSts
  Logical Operator : Logic  Operator=OR  AllPortsSameDT=off  OutDataTypeStr=boolean
  NTC Sts Calculation : Subsystem
  Relational Operator1 : RelationalOperator  Operator=<  OutDataTypeStr=boolean
  Relational Operator2 : RelationalOperator  Operator=<  OutDataTypeStr=boolean
  Switch Case1 : SwitchCase  CaseConditions={StHlthMonSig3.STHLTHMONSIG_CURRMOTSUMABC}
  CurrMotSumDEFStHlth : Outport
  CurrMotSumABCStHlth : Outport  Port=2
  wires:
  Constant3/1 -> CurrMotSumPhaStHlth/1(NtcNr)
  Constant1/1 -> CurrMotSumPhaStHlth/2(NtcStInfo)
  Constant5/1 -> CurrMotSumPhaStHlth/4(DebStep)
  NTC Sts Calculation/1(NtcSts) -> CurrMotSumPhaStHlth/3(NtcSts)
  Switch Case1/1 -> CurrMotSumABCStHlth Calc/Action
  Switch Case1/2 -> CurrMotSumDEFStHlth Calc/Action
  CurrMotSumDEF/1 -> CurrMotSumDEFStHlth Calc/1(CurrMotSumDEF)
  CurrMotSumABC/1 -> CurrMotSumABCStHlth Calc/1(CurrMotSumABC)
  CurrMotSumABCStHlth Calc/1(CurrMotSumABCStHlth) -> Data Store Write/1, CurrMotSumABCStHlth/1
  CurrMotSumDEFStHlth Calc/1(CurrMotSumDEFStHlth) -> Data Store Write1/1, CurrMotSumDEFStHlth/1
  SigId/1 -> Switch Case1/1
  Constant2/1 -> Relational Operator2/2
  Relational Operator2/1 -> Logical Operator/1
  Data Store Read/1 -> Relational Operator2/1
  Constant4/1 -> Relational Operator1/2
  Relational Operator1/1 -> Logical Operator/2
  Data Store Read1/1 -> Relational Operator1/1
  Logical Operator/1 -> NTC Sts Calculation/1(StHlthErr)

== system ES105A_StHlthSigNormn/StHlthSigNormn/UpdRawSig/Default ==
  note: This is a default case.
      |
      | No data processing will be done.
  "Case:{}" : ActionPort  ActionType=default
  CopyRight2 : Subsystem  Description=|  mask(Copyright Information){none=on}
      | Copyright info block.                                               
      |                                                                     
      | Place copyright information at the top of every subsystem in design.
      mask prompts: none "No parameters"
      mask help: Place copyright information at the top of every subsystem in design.
      mask Display:
      | NxtrConf = 'Nexteer Confidential';
      | 
      | sys = bdroot; %handle for the current model ("system")
      | first = get_param(sys,'Created');
      | first = first(end-3:end);  %year is last four digits
      | 
      | last = get_param(sys,'LastModifiedDate');
      | if isempty(last)
      |     last = datestr(now,'yyyy');
      | else
      |     last = last(end-3:end);
      | end
      | 
      | if strcmp(first,last)
      |     fprintf('%s -- Copyright %s Nexteer',NxtrConf,first)
      | else
      |     fprintf('%s -- %s%s- %s Nexteer',NxtrConf,char(169),first,last)
      | end

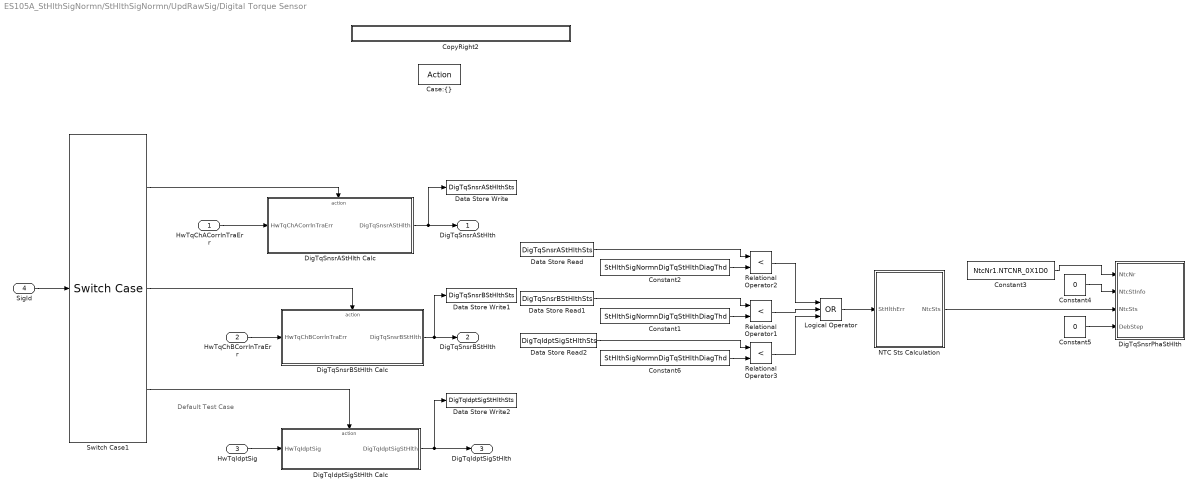
== system ES105A_StHlthSigNormn/StHlthSigNormn/UpdRawSig/Digital Torque Sensor  ==
  note: Default Test Case
  HwTqChACorrlnTraErr : Inport
  HwTqChBCorrlnTraErr : Inport  Port=2
  HwTqIdptSig : Inport  Port=3
  SigId : Inport  Port=4
  "Case:{}" : ActionPort  ActionType=case
  Constant1 : Constant  Value=StHlthSigNormnDigTqStHlthDiagThd
  Constant2 : Constant  Value=StHlthSigNormnDigTqStHlthDiagThd
  Constant3 : Constant  Value=NtcNr1.NTCNR_0X1D0  OutDataTypeStr=Enum: NtcNr1
  Constant4 : Constant  Value=0  OutDataTypeStr=uint8
      settings: AttributesFormatString=%<OutDataTypeStr>
  Constant5 : Constant  Value=0  OutDataTypeStr=uint16
      settings: AttributesFormatString=%<OutDataTypeStr>
  Constant6 : Constant  Value=StHlthSigNormnDigTqStHlthDiagThd
  CopyRight2 : Subsystem  Description=|  mask(Copyright Information){none=on}
      | Copyright info block.                                               
      |                                                                     
      | Place copyright information at the top of every subsystem in design.
      mask prompts: none "No parameters"
      mask help: Place copyright information at the top of every subsystem in design.
      mask Display:
      | NxtrConf = 'Nexteer Confidential';
      | 
      | sys = bdroot; %handle for the current model ("system")
      | first = get_param(sys,'Created');
      | first = first(end-3:end);  %year is last four digits
      | 
      | last = get_param(sys,'LastModifiedDate');
      | if isempty(last)
      |     last = datestr(now,'yyyy');
      | else
      |     last = last(end-3:end);
      | end
      | 
      | if strcmp(first,last)
      |     fprintf('%s -- Copyright %s Nexteer',NxtrConf,first)
      | else
      |     fprintf('%s -- %s%s- %s Nexteer',NxtrConf,char(169),first,last)
      | end
  Data Store Read : DataStoreRead  DataStoreName=DigTqSnsrAStHlthSts
  Data Store Read1 : DataStoreRead  DataStoreName=DigTqSnsrBStHlthSts
  Data Store Read2 : DataStoreRead  DataStoreName=DigTqIdptSigStHlthSts
  Data Store Write : DataStoreWrite  DataStoreName=DigTqSnsrAStHlthSts
  Data Store Write1 : DataStoreWrite  DataStoreName=DigTqSnsrBStHlthSts
  Data Store Write2 : DataStoreWrite  DataStoreName=DigTqIdptSigStHlthSts
  DigTqIdptSigStHlth Calc : Subsystem  TreatAsAtomicUnit=on
  DigTqSnsrAStHlth Calc : Subsystem  TreatAsAtomicUnit=on
  DigTqSnsrBStHlth Calc : Subsystem  TreatAsAtomicUnit=on
  DigTqSnsrPhaStHlth : Subsystem  mask(SetNTC){}
      mask help: SetNTC library block
  Logical Operator : Logic  Operator=OR  Inputs=3  AllPortsSameDT=off  OutDataTypeStr=boolean
  NTC Sts Calculation : Subsystem
  Relational Operator1 : RelationalOperator  Operator=<  OutDataTypeStr=boolean
  Relational Operator2 : RelationalOperator  Operator=<  OutDataTypeStr=boolean
  Relational Operator3 : RelationalOperator  Operator=<  OutDataTypeStr=boolean
  Switch Case1 : SwitchCase  CaseConditions={StHlthMonSig3.STHLTHMONSIG_DIGTQSNSRA,StHlthMonSig3.STHLTHMONSIG_DIGTQSNSRB}
  DigTqSnsrAStHlth : Outport
  DigTqSnsrBStHlth : Outport  Port=2
  " DigTqIdptSigStHlth" : Outport  Port=3
  wires:
  SigId/1 -> Switch Case1/1
  Switch Case1/1 -> DigTqSnsrAStHlth Calc/Action
  Switch Case1/2 -> DigTqSnsrBStHlth Calc/Action
  Switch Case1/3 -> DigTqIdptSigStHlth Calc/Action
  HwTqChACorrlnTraErr/1 -> DigTqSnsrAStHlth Calc/1(HwTqChACorrlnTraErr)
  HwTqChBCorrlnTraErr/1 -> DigTqSnsrBStHlth Calc/1(HwTqChBCorrlnTraErr)
  HwTqIdptSig/1 -> DigTqIdptSigStHlth Calc/1(HwTqIdptSig)
  DigTqSnsrAStHlth Calc/1(DigTqSnsrAStHlth) -> Data Store Write/1, DigTqSnsrAStHlth/1
  DigTqIdptSigStHlth Calc/1(" DigTqIdptSigStHlth") -> Data Store Write2/1, " DigTqIdptSigStHlth"/1
  DigTqSnsrBStHlth Calc/1(DigTqSnsrBStHlth) -> Data Store Write1/1, DigTqSnsrBStHlth/1
  Constant3/1 -> DigTqSnsrPhaStHlth/1(NtcNr)
  Constant4/1 -> DigTqSnsrPhaStHlth/2(NtcStInfo)
  Constant5/1 -> DigTqSnsrPhaStHlth/4(DebStep)
  Constant2/1 -> Relational Operator2/2
  Data Store Read/1 -> Relational Operator2/1
  Constant1/1 -> Relational Operator1/2
  Data Store Read1/1 -> Relational Operator1/1
  Constant6/1 -> Relational Operator3/2
  Data Store Read2/1 -> Relational Operator3/1
  Relational Operator2/1 -> Logical Operator/1
  Relational Operator1/1 -> Logical Operator/2
  Relational Operator3/1 -> Logical Operator/3
  Logical Operator/1 -> NTC Sts Calculation/1(StHlthErr)
  NTC Sts Calculation/1(NtcSts) -> DigTqSnsrPhaStHlth/3(NtcSts)

== system ES105A_StHlthSigNormn/StHlthSigNormn/UpdRawSig/Duty Cycle Exceeded ==
  DutyCycThermProtnMaxOutp : Inport
  "Case:{}" : ActionPort  ActionType=case
  Constant : Constant  Value=DutyCycThermProtnDutyCycFildThd
  Constant1 : Constant  Value=StHlthSigNormnDutyCycFltLimThd
  CopyRight2 : Subsystem  Description=|  mask(Copyright Information){none=on}
      | Copyright info block.                                               
      |                                                                     
      | Place copyright information at the top of every subsystem in design.
      mask prompts: none "No parameters"
      mask help: Place copyright information at the top of every subsystem in design.
      mask Display:
      | NxtrConf = 'Nexteer Confidential';
      | 
      | sys = bdroot; %handle for the current model ("system")
      | first = get_param(sys,'Created');
      | first = first(end-3:end);  %year is last four digits
      | 
      | last = get_param(sys,'LastModifiedDate');
      | if isempty(last)
      |     last = datestr(now,'yyyy');
      | else
      |     last = last(end-3:end);
      | end
      | 
      | if strcmp(first,last)
      |     fprintf('%s -- Copyright %s Nexteer',NxtrConf,first)
      | else
      |     fprintf('%s -- %s%s- %s Nexteer',NxtrConf,char(169),first,last)
      | end
  If : If  NumInputs=2  IfExpression=u1  ElseIfExpressions=u2
  If Action Subsystem : Subsystem  TreatAsAtomicUnit=on
  If Action Subsystem1 : Subsystem  TreatAsAtomicUnit=on
  If Action Subsystem2 : Subsystem  TreatAsAtomicUnit=on
  LimStat_u2 : NxtrLim/LimStat_u08  LoLim=DutyCycStHlth.EngMin  HiLim=DutyCycStHlth.EngMax
      settings: AttributesFormatString=|
      | Low Limit: %<LoLim>
      | High Limit:%<HiLim>
  Merge : Merge  Inputs=3
  Relational Operator : RelationalOperator  OutDataTypeStr=boolean
  Relational Operator1 : RelationalOperator  OutDataTypeStr=boolean
  DutyCycStHlth : Outport
  wires:
  Constant/1 -> Relational Operator/2
  Relational Operator/1 -> If/1
  If/1 -> If Action Subsystem/Action
  DutyCycThermProtnMaxOutp/1 -> Relational Operator1/1, Relational Operator/1
  Constant1/1 -> Relational Operator1/2
  Relational Operator1/1 -> If/2
  If/3 -> If Action Subsystem2/Action
  If/2 -> If Action Subsystem1/Action
  If Action Subsystem/1(DutyCycStHlth) -> Merge/1
  If Action Subsystem1/1(DutyCycStHlth) -> Merge/2
  If Action Subsystem2/1(DutyCycStHlth) -> Merge/3
  Merge/1 -> LimStat_u2/1
  LimStat_u2/1 -> DutyCycStHlth/1

== system ES105A_StHlthSigNormn/StHlthSigNormn/UpdRawSig/Friction Estimation ==
  note: Merge block was highlighted as
      | we can't highlight a line alone.
  MaxLrndFric : Inport
  EOLFric : Inport  Port=2
  "Case:{}" : ActionPort  ActionType=case
  Constant4 : Constant  Value=StHlthSigNormnMaxFricThd
  CopyRight2 : Subsystem  Description=|  mask(Copyright Information){none=on}
      | Copyright info block.                                               
      |                                                                     
      | Place copyright information at the top of every subsystem in design.
      mask prompts: none "No parameters"
      mask help: Place copyright information at the top of every subsystem in design.
      mask Display:
      | NxtrConf = 'Nexteer Confidential';
      | 
      | sys = bdroot; %handle for the current model ("system")
      | first = get_param(sys,'Created');
      | first = first(end-3:end);  %year is last four digits
      | 
      | last = get_param(sys,'LastModifiedDate');
      | if isempty(last)
      |     last = datestr(now,'yyyy');
      | else
      |     last = last(end-3:end);
      | end
      | 
      | if strcmp(first,last)
      |     fprintf('%s -- Copyright %s Nexteer',NxtrConf,first)
      | else
      |     fprintf('%s -- %s%s- %s Nexteer',NxtrConf,char(169),first,last)
      | end
  If Action Subsystem3 : Subsystem  TreatAsAtomicUnit=on
  If Action Subsystem4 : Subsystem  TreatAsAtomicUnit=on
  If1 : If  IfExpression=u1
  Merge : Merge
  Relational Operator4 : RelationalOperator  Operator=<=  OutDataTypeStr=boolean
  FricEstimnStHlth : Outport
  wires:
  Merge/1 -> FricEstimnStHlth/1
  Constant4/1 -> Relational Operator4/2
  Relational Operator4/1 -> If1/1
  MaxLrndFric/1 -> [MaxLrndFric], Relational Operator4/1
  If Action Subsystem3/1(FricEstStHlth) -> Merge/2
  If1/2 -> If Action Subsystem3/Action
  If1/1 -> If Action Subsystem4/Action
  If Action Subsystem4/1(FricEstStHlth) -> Merge/1
  [MaxLrndFric] -> If Action Subsystem4/1(MaxLrndFric)
  EOLFric/1 -> If Action Subsystem4/2(EOLFric)

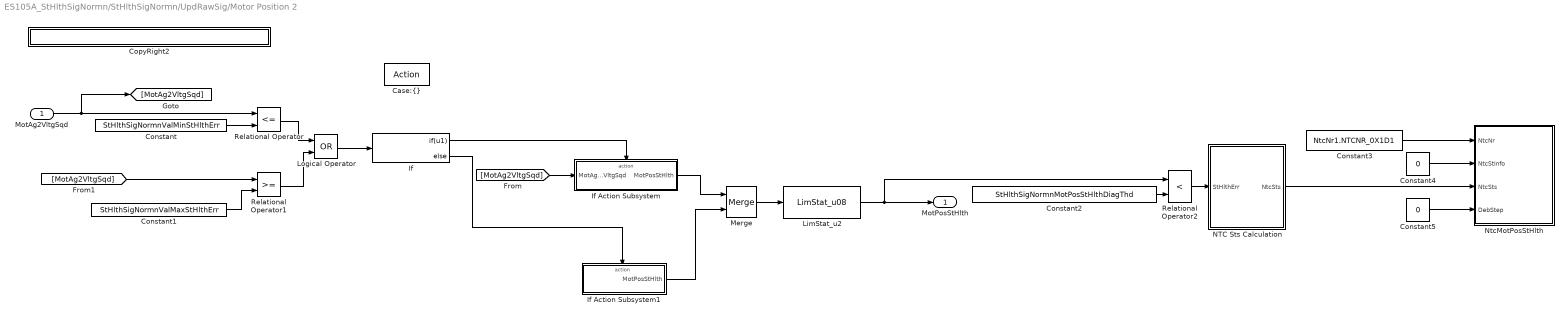
== system ES105A_StHlthSigNormn/StHlthSigNormn/UpdRawSig/Motor Position 2  ==
  MotAg2VltgSqd : Inport
  "Case:{}" : ActionPort  ActionType=case
  Constant : Constant  Value=StHlthSigNormnValMinStHlthErr
  Constant1 : Constant  Value=StHlthSigNormnValMaxStHlthErr
  Constant2 : Constant  Value=StHlthSigNormnMotPosStHlthDiagThd
  Constant3 : Constant  Value=NtcNr1.NTCNR_0X1D1  OutDataTypeStr=Enum: NtcNr1
  Constant4 : Constant  Value=0  OutDataTypeStr=uint8
      settings: AttributesFormatString=%<OutDataTypeStr>
  Constant5 : Constant  Value=0  OutDataTypeStr=uint16
      settings: AttributesFormatString=%<OutDataTypeStr>
  CopyRight2 : Subsystem  Description=|  mask(Copyright Information){none=on}
      | Copyright info block.                                               
      |                                                                     
      | Place copyright information at the top of every subsystem in design.
      mask prompts: none "No parameters"
      mask help: Place copyright information at the top of every subsystem in design.
      mask Display:
      | NxtrConf = 'Nexteer Confidential';
      | 
      | sys = bdroot; %handle for the current model ("system")
      | first = get_param(sys,'Created');
      | first = first(end-3:end);  %year is last four digits
      | 
      | last = get_param(sys,'LastModifiedDate');
      | if isempty(last)
      |     last = datestr(now,'yyyy');
      | else
      |     last = last(end-3:end);
      | end
      | 
      | if strcmp(first,last)
      |     fprintf('%s -- Copyright %s Nexteer',NxtrConf,first)
      | else
      |     fprintf('%s -- %s%s- %s Nexteer',NxtrConf,char(169),first,last)
      | end
  If : If  IfExpression=u1
  If Action Subsystem : Subsystem  TreatAsAtomicUnit=on
  If Action Subsystem1 : Subsystem  TreatAsAtomicUnit=on
  LimStat_u2 : NxtrLim/LimStat_u08  LoLim=MotPosStHlth.EngMin  HiLim=MotPosStHlth.EngMax
      settings: AttributesFormatString=|
      | Low Limit: %<LoLim>
      | High Limit:%<HiLim>
  Logical Operator : Logic  Operator=OR  AllPortsSameDT=off  OutDataTypeStr=boolean
  Merge : Merge
  NTC Sts Calculation : Subsystem
  NtcMotPosStHlth : Subsystem  mask(SetNTC){}
      mask help: SetNTC library block
  Relational Operator : RelationalOperator  Operator=<=  OutDataTypeStr=boolean
  Relational Operator1 : RelationalOperator  OutDataTypeStr=boolean
  Relational Operator2 : RelationalOperator  Operator=<  OutDataTypeStr=boolean
  MotPosStHlth : Outport
  wires:
  Constant/1 -> Relational Operator/2
  MotAg2VltgSqd/1 -> Relational Operator/1, [MotAg2VltgSqd]
  Constant1/1 -> Relational Operator1/2
  Relational Operator/1 -> Logical Operator/1
  Relational Operator1/1 -> Logical Operator/2
  Logical Operator/1 -> If/1
  If/1 -> If Action Subsystem/Action
  If/2 -> If Action Subsystem1/Action
  If Action Subsystem/1(MotPosStHlth) -> Merge/1
  If Action Subsystem1/1(MotPosStHlth) -> Merge/2
  Merge/1 -> LimStat_u2/1
  [MotAg2VltgSqd] -> If Action Subsystem/1(MotAg2VltgSqd)
  Constant3/1 -> NtcMotPosStHlth/1(NtcNr)
  Constant4/1 -> NtcMotPosStHlth/2(NtcStInfo)
  Constant5/1 -> NtcMotPosStHlth/4(DebStep)
  [MotAg2VltgSqd] -> Relational Operator1/1
  Constant2/1 -> Relational Operator2/2
  LimStat_u2/1 -> Relational Operator2/1, MotPosStHlth/1
  Relational Operator2/1 -> NTC Sts Calculation/1(StHlthErr)
  NTC Sts Calculation/1(NtcSts) -> NtcMotPosStHlth/3(NtcSts)
